simulink model "ClosedLoopSecondOrder"  (R2021a)
settings: Solver=VariableStepAuto  StartTime=0.0  StopTime=10.0  RelTol=1e-3
settings Model: Creator=soumy  LastModifiedBy=soumy

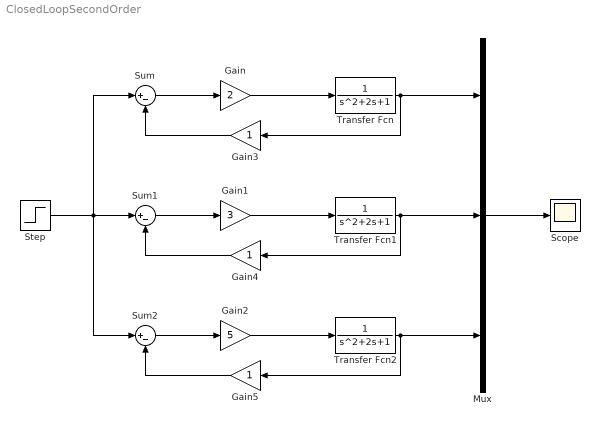
== system ClosedLoopSecondOrder ==
  Gain : Gain  Gain=2
  Gain1 : Gain  Gain=3
  Gain2 : Gain  Gain=5
  Gain3 : Gain
  Gain4 : Gain
  Gain5 : Gain
  Mux : Mux  Inputs=3
  Scope : Scope
  Step : Step  SampleTime=0
  Sum : Sum  Inputs=|+-
  Sum1 : Sum  Inputs=|+-
  Sum2 : Sum  Inputs=|+-
  Transfer Fcn : TransferFcn
  Transfer Fcn1 : TransferFcn
  Transfer Fcn2 : TransferFcn
  wires:
  Mux/1 -> Scope/1
  Gain/1 -> Transfer Fcn/1
  Gain1/1 -> Transfer Fcn1/1
  Gain2/1 -> Transfer Fcn2/1
  Transfer Fcn2/1 -> Gain5/1, Mux/3
  Transfer Fcn/1 -> Gain3/1, Mux/1
  Transfer Fcn1/1 -> Gain4/1, Mux/2
  Step/1 -> Sum1/1, Sum2/1, Sum/1
  Gain4/1 -> Sum1/2
  Sum/1 -> Gain/1
  Gain3/1 -> Sum/2
  Sum1/1 -> Gain1/1
  Gain5/1 -> Sum2/2
  Sum2/1 -> Gain2/1
